simulink model "heli_q8_4_emmerich"  (R2020b)
settings: Solver=ode1  StartTime=0.0  StopTime=inf  FixedStep=0.002  RelTol=1e-3  EnableMultiTasking=on
PostLoadFcn:
  | qc_set_target_type(getConfigSet(bdroot, 'QUARC Default Target Configuration'));
values from neighbouring files (symbols this model uses):
  Ad = eye(6) + T*A + 1/factorial(2)*T^2*A^2 + 1/factorial(3)*T^3*A^3    [init_lab_4.m]
  Bd = (T*eye(6) + 1/factorial(2)*A*T^2 + 1/factorial(3)*A^2*T^3 + 1/factorial(4)*A^3*T^4)*B    [init_lab_4.m]
  Cd = [1 0 0 0 0 0 ... (first row only)    [init_lab_4.m]
  P_init = zeros(6)    [init_lab_4.m]
  Qd = 1000*eye(6)    [init_lab_4.m]
  Rd_move = cov(data_move')    [init_lab_4.m]
  x_init = zeros(6, 1)    [init_lab_4.m]
undefined symbols (not defined in the file or in its folder): F, HIL, Joystick_gain_x, Joystick_gain_y, K, qc_get_step_size, vs0
libraries: quarc_library x9
settings Model: SimulationMode=external  ExtModeTrigDuration=5000  Creator=Rchan  LastModifiedBy=tadyrkor
settings SolverCC: PositivePriorityOrder=on
settings DataIOCC: LimitDataPoints=on  SaveFormat=Array  SignalLoggingSaveFormat=ModelDataLogs  ReturnWorkspaceOutputs=off
settings OptimizationCC: ExpressionDepthLimit=2147483647  InitFltsAndDblsToZero=on  LifeSpan=inf
settings DebuggingCC: SaveWithParameterizedLinksMsg=none  UnderspecifiedInitializationDetection=Classic  MergeDetectMultiDrivingBlocksExec=none  SolverPrmCheckMsg=warning  MultiTaskDSMMsg=warning  MultiTaskCondExecSysMsg=none  FcnCallInpInsideContextMsg=warning  AllowSymbolicDim=off  StateNameClashWarn=warning  SFUnexpectedBacktrackingDiag=warning  SFNoUnconditionalDefaultTransitionDiag=warning  SFExecutionAtInitializationDiag=none  ArithmeticOperatorsInVariantConditions=warning
settings HardwareCC: ProdBitPerPointer=32  ProdBitPerSizeT=32  ProdBitPerPtrDiffT=32  ProdLargestAtomicFloat=None  ProdIntDivRoundTo=Undefined  ProdEndianess=Unspecified  ProdWordSize=32  ProdHWDeviceType=32-bit Generic
settings ModelReferenceCC: PropagateSignalLabelsOutOfModel=off
settings SFSimCC: SimUseLocalCustomCode=off  CustomCodeUndefinedFunction=UseInterfaceOnly
settings RTWCC: Description=QUARC Win64 Target  SystemTargetFile=quarc_win64.tlc  TemplateMakefile=quarc_default_tmf  RTWUseLocalCustomCode=off
settings CodeAppCC: StateflowObjectComments=on
settings GRTTargetCC: TargetLangStandard=C89/C90 (ANSI)  ParMdlRefBuildCompliant=off  CompOptLevelCompliant=off  CombineOutputUpdateFcns=off  MatFileLogging=off  GRTInterface=on  UseToolchainInfoCompliant=off  ExtMode=on  ExtModeMexFile=quarc_comm
settings ConfigComp: CovMetricSettings=dw  CovSaveCumulativeToWorkspaceVar=on  CovSaveSingleToWorkspaceVar=on  CovExternalEMLEnable=off  CovSFcnEnable=off

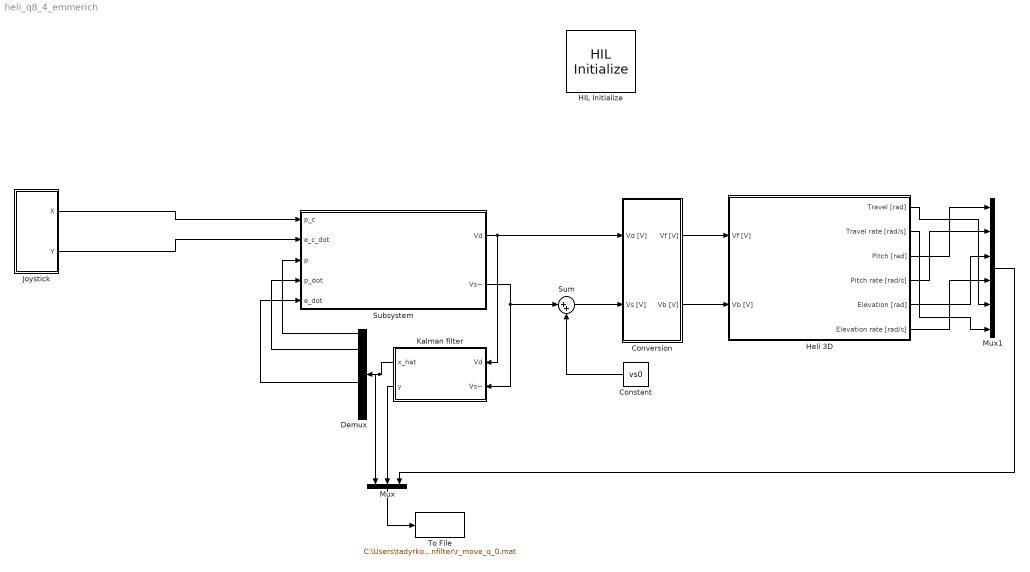
== system heli_q8_4_emmerich ==
  Constant : Constant  Value=vs0
  Conversion : Subsystem
  Demux : Demux  Outputs=6
  HIL Initialize : quarc_library/Data Acquisition/Generic/Configuration/HIL Initialize  Priority=-99  object_name=HIL-1  board_type=q8_usb  board_number=0  board_options=update_rate=normal;decimation=1  exclusive=off  active=off  hardware_clocks=[0:2]  clock_modes=[]  initial_clock_frequencies=[]  set_clock_params_at_start=off  set_clock_params_at_switch_in=off  set_clock_frequencies_at_start=off  set_clock_frequencies_at_switch_in=off  analog_input_channels=[0:7]  analog_input_configurations=[]  analog_input_maximums=10  analog_input_minimums=-10  set_analog_input_params_at_start=on  set_analog_input_params_at_switch_in=off  analog_output_channels=[0:7]  analog_output_maximums=10  analog_output_minimums=-10  initial_analog_outputs=[0]  final_analog_outputs=[0]  watchdog_analog_outputs=0  set_analog_output_params_at_start=on  set_analog_output_params_at_switch_in=off  set_analog_outputs_at_start=on  set_analog_outputs_at_switch_in=off  set_analog_outputs_at_terminate=on  set_analog_outputs_at_switch_out=off  set_analog_outputs_on_watchdog=off  digital_input_channels=[]  digital_output_channels=[]  digital_output_configuration=[]  initial_digital_outputs=[1]  final_digital_outputs=[1]  watchdog_digital_outputs=[1]  set_digital_output_params_at_start=off  set_digital_output_params_at_switch_in=off  set_digital_outputs_at_start=on  set_digital_outputs_at_switch_in=off  set_digital_outputs_at_terminate=on  set_digital_outputs_at_switch_out=off  set_digital_outputs_on_watchdog=off  encoder_channels=[0:7]  quadrature=[4]  encoder_filter_frequency=[]  initial_encoder_counts=[0]  set_encoder_params_at_start=on  set_encoder_params_at_switch_in=off  set_encoder_counts_at_start=on  set_encoder_counts_at_switch_in=off  pwm_channels=[0:7]  pwm_modes=0  pwm_frequency=99.532799999999995e6/4095  pwm_configuration=[0]  pwm_alignment=[0]  pwm_polarity=[1]  pwm_leading_deadband=[0]  pwm_trailing_deadband=[0]  initial_pwm_outputs=[0]  final_pwm_outputs=[0]  watchdog_pwm_outputs=[0]  set_pwm_params_at_start=on  set_pwm_params_at_switch_in=off  set_pwm_outputs_at_start=on  set_pwm_outputs_at_switch_in=off  set_pwm_outputs_at_terminate=on  set_pwm_outputs_at_switch_out=off  set_pwm_outputs_on_watchdog=off  other_output_channels=[]  initial_other_outputs=[]  final_other_outputs=[]  watchdog_other_outputs=[]  set_other_outputs_at_start=off  set_other_outputs_at_switch_in=off  set_other_outputs_at_terminate=off  set_other_outputs_at_switch_out=off  set_other_outputs_on_watchdog=off
  Heli 3D : Subsystem
  Joystick : Subsystem
  Kalman filter : Subsystem
  Mux : Mux  Inputs=3
  Mux1 : Mux  Inputs=6
  Subsystem : Subsystem
  Sum : Sum  Inputs=|++
  To File : ToFile  Filename=C:\Users\tadyrkor\Documents\data\lab4\kalmanfilter\r_move_q_0.mat  MatrixName=measurements
  wires:
  Conversion/2(Vb [V]) -> Heli 3D/2(Vb [V])
  Conversion/1(Vf [V]) -> Heli 3D/1(Vf [V])
  Subsystem/2(Vs~) -> Sum/1, Kalman filter/2(Vs~)
  Subsystem/1(Vd) -> Conversion/1(Vd [V]), Kalman filter/1(Vd)
  Joystick/1(X) -> Subsystem/1(p_c)
  Joystick/2(Y) -> Subsystem/2(e_c_dot)
  Constant/1 -> Sum/2
  Sum/1 -> Conversion/2(Vs [V])
  Kalman filter/1(x_hat) -> Mux/1, Demux/1
  Demux/1 -> Subsystem/3(p)
  Demux/2 -> Subsystem/4(p_dot)
  Demux/4 -> Subsystem/5(e_dot)
  Kalman filter/2(y) -> Mux/2
  Heli 3D/3(Pitch [rad]) -> Mux1/1
  Heli 3D/4(Pitch rate [rad/s]) -> Mux1/2
  Heli 3D/5(Elevation [rad]) -> Mux1/3
  Heli 3D/6(Elevation rate [rad/s]) -> Mux1/4
  Heli 3D/1(Travel [rad]) -> Mux1/5
  Heli 3D/2(Travel rate [rad/s]) -> Mux1/6
  Mux1/1 -> Mux/3
  Mux/1 -> To File/1

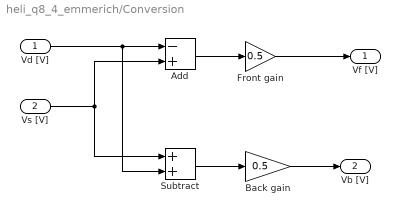
== system heli_q8_4_emmerich/Conversion ==
  Vd [V] : Inport
  Vs [V] : Inport  Port=2
  Add : Sum  Inputs=-+
  Back gain : Gain  Gain=0.5
  Front gain : Gain  Gain=0.5
  Subtract : Sum
  Vf [V] : Outport
  Vb [V] : Outport  Port=2
  wires:
  Vd [V]/1 -> Subtract/2, Add/1
  Vs [V]/1 -> Subtract/1, Add/2
  Subtract/1 -> Back gain/1
  Back gain/1 -> Vb [V]/1
  Add/1 -> Front gain/1
  Front gain/1 -> Vf [V]/1

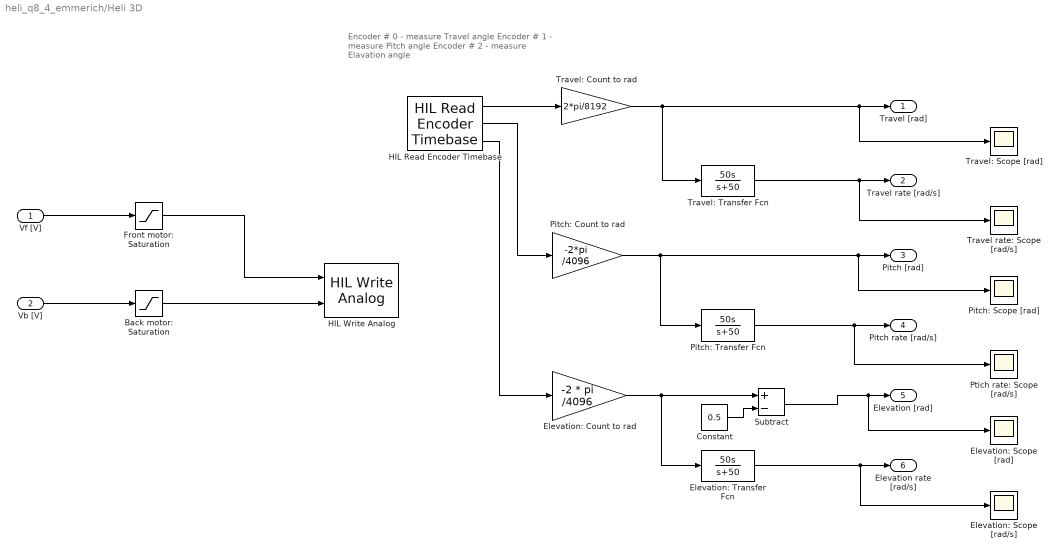
== system heli_q8_4_emmerich/Heli 3D ==
  note: Encoder # 0 - measure Travel angle
      | Encoder # 1 - measure Pitch angle
      | Encoder # 2 - measure Elavation angle
  Vf [V] : Inport
  Vb [V] : Inport  Port=2
  Back motor: Saturation : Saturate  UpperLimit=5  LowerLimit=-5
  Constant : Constant  Value=0.5
  Elevation: Count to rad : Gain  Gain=-2 * pi /4096
  Elevation: Scope [rad/s] : Scope
  Elevation: Scope [rad] : Scope
  Elevation: Transfer Fcn : TransferFcn  Numerator=[50 0]  Denominator=[1 50]
  Front motor: Saturation : Saturate  UpperLimit=5  LowerLimit=-5
  HIL Read Encoder Timebase : quarc_library/Data Acquisition/Generic/Timebases/HIL Read Encoder Timebase  object_name=HIL-1  clock=0  channels=[0:2]  active=on  vector_output=off  data_type_mode=Inherit via back propagation  data_type=double  overflow_mode=Error on overflow  samples_in_buffer=max(ceil(1/qc_get_step_size), 1)
  HIL Write Analog : quarc_library/Data Acquisition/Generic/Immediate I//O/HIL Write Analog  object_name=HIL-1  channels=[0:1]  sample_time=-1  active=off  vector_input=off
  Pitch: Count to rad : Gain  Gain=-2*pi /4096
  Pitch: Scope [rad] : Scope
  Pitch: Transfer Fcn : TransferFcn  Numerator=[50 0]  Denominator=[1 50]
  Ptich rate: Scope [rad/s] : Scope
  Subtract : Sum  Inputs=+-
  Travel rate: Scope [rad/s] : Scope
  Travel: Count to rad : Gain  Gain=2*pi/8192
  Travel: Scope [rad] : Scope
  Travel: Transfer Fcn : TransferFcn  Numerator=[50 0]  Denominator=[1 50]
  Travel [rad] : Outport
  Travel rate [rad/s] : Outport  Port=2
  Pitch [rad] : Outport  Port=3
  Pitch rate [rad/s] : Outport  Port=4
  Elevation [rad] : Outport  Port=5
  Elevation rate [rad/s] : Outport  Port=6
  wires:
  HIL Read Encoder Timebase/1 -> Travel: Count to rad/1
  HIL Read Encoder Timebase/2 -> Pitch: Count to rad/1
  HIL Read Encoder Timebase/3 -> Elevation: Count to rad/1
  Travel: Count to rad/1 -> Travel: Scope [rad]/1, Travel [rad]/1, Travel: Transfer Fcn/1
  Travel: Transfer Fcn/1 -> Travel rate: Scope [rad/s]/1, Travel rate [rad/s]/1
  Pitch: Count to rad/1 -> Pitch: Transfer Fcn/1, Pitch: Scope [rad]/1, Pitch [rad]/1
  Pitch: Transfer Fcn/1 -> Ptich rate: Scope [rad/s]/1, Pitch rate [rad/s]/1
  Elevation: Count to rad/1 -> Subtract/1, Elevation: Transfer Fcn/1
  Elevation: Transfer Fcn/1 -> Elevation: Scope [rad/s]/1, Elevation rate [rad/s]/1
  Vf [V]/1 -> Front motor: Saturation/1
  Vb [V]/1 -> Back motor: Saturation/1
  Front motor: Saturation/1 -> HIL Write Analog/1
  Back motor: Saturation/1 -> HIL Write Analog/2
  Subtract/1 -> Elevation: Scope [rad]/1, Elevation [rad]/1
  Constant/1 -> Subtract/2

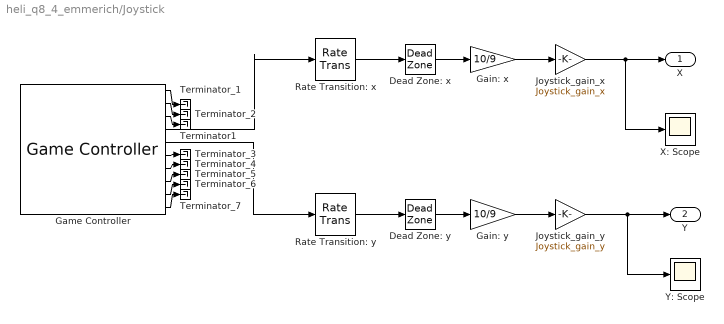
== system heli_q8_4_emmerich/Joystick ==
  Dead Zone: x : DeadZone  LowerValue=-0.1  UpperValue=0.1  SaturateOnIntegerOverflow=on
  Dead Zone: y : DeadZone  LowerValue=-0.1  UpperValue=0.1  SaturateOnIntegerOverflow=on
  Gain: x : Gain  Gain=10/9
  Gain: y : Gain  Gain=10/9
  Game Controller : quarc_library/Devices/Peripherals/Target/Game Controller  controller=1  buffer_size=12  deadzone=[]  saturation=[]  sample_time=max(qc_get_step_size, 0.01)  auto_center=off  enabled=on
      settings: SourceProductName=QUARC Targets
  Joystick_gain_x : Gain  Gain=Joystick_gain_x
  Joystick_gain_y : Gain  Gain=Joystick_gain_y
  Rate Transition: x : RateTransition
  Rate Transition: y : RateTransition
  Terminator1 : Terminator
  Terminator_{1..7} (7 alike) : Terminator
  X: Scope : Scope
  Y: Scope : Scope
  X : Outport
  Y : Outport  Port=2
  wires:
  Rate Transition: y/1 -> Dead Zone: y/1
  Rate Transition: x/1 -> Dead Zone: x/1
  Game Controller/5 -> Rate Transition: y/1
  Game Controller/4 -> Rate Transition: x/1
  Game Controller/1 -> Terminator_1/1
  Game Controller/2 -> Terminator_2/1
  Game Controller/7 -> Terminator_4/1
  Game Controller/8 -> Terminator_5/1
  Game Controller/9 -> Terminator_6/1
  Game Controller/10 -> Terminator_7/1
  Game Controller/3 -> Terminator1/1
  Dead Zone: x/1 -> Gain: x/1
  Dead Zone: y/1 -> Gain: y/1
  Gain: x/1 -> Joystick_gain_x/1
  Gain: y/1 -> Joystick_gain_y/1
  Joystick_gain_x/1 -> X/1, X: Scope/1
  Joystick_gain_y/1 -> Y: Scope/1, Y/1
  Game Controller/6 -> Terminator_3/1

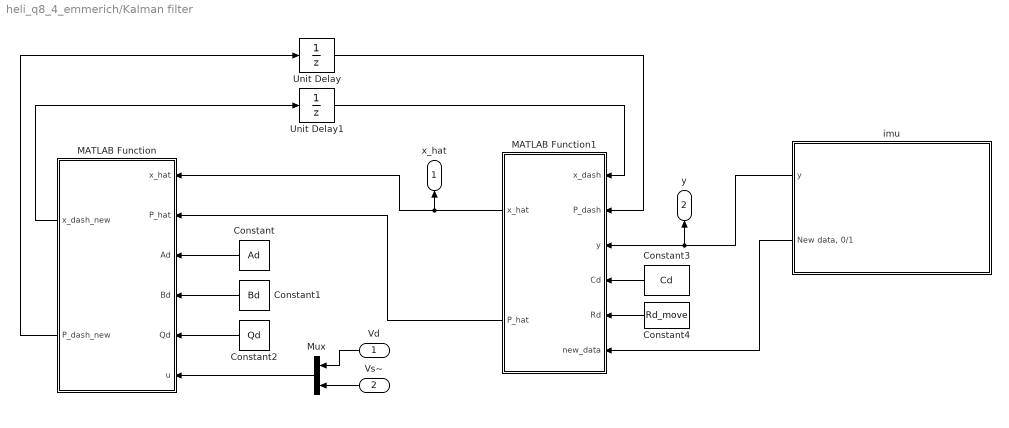
== system heli_q8_4_emmerich/Kalman filter ==
  Vd : Inport
  Vs~ : Inport  Port=2
  Constant : Constant  Value=Ad
  Constant1 : Constant  Value=Bd
  Constant2 : Constant  Value=Qd
  Constant3 : Constant  Value=Cd
  Constant4 : Constant  Value=Rd_move
  MATLAB Function : MATLAB Function  TreatAsAtomicUnit=on
  MATLAB Function1 : MATLAB Function  TreatAsAtomicUnit=on
  Mux : Mux  Inputs=2
  Unit Delay : UnitDelay  InitialCondition=P_init  SampleTime=-1  HasFrameUpgradeWarning=on
  Unit Delay1 : UnitDelay  InitialCondition=x_init  SampleTime=-1  HasFrameUpgradeWarning=on
  imu : Subsystem
  x_hat : Outport
  y : Outport  Port=2
  wires:
  Vs~/1 -> Mux/2
  Vd/1 -> Mux/1
  Mux/1 -> MATLAB Function/6(u)
  imu/1(y) -> MATLAB Function1/3(y), y/1
  imu/2("New data, 0/1") -> MATLAB Function1/6(new_data)
  MATLAB Function1/2(P_hat) -> MATLAB Function/2(P_hat)
  Constant/1 -> MATLAB Function/3(Ad)
  Constant2/1 -> MATLAB Function/5(Qd)
  Constant1/1 -> MATLAB Function/4(Bd)
  Constant3/1 -> MATLAB Function1/4(Cd)
  Constant4/1 -> MATLAB Function1/5(Rd)
  MATLAB Function/1(x_dash_new) -> Unit Delay1/1
  MATLAB Function/2(P_dash_new) -> Unit Delay/1
  Unit Delay/1 -> MATLAB Function1/2(P_dash)
  Unit Delay1/1 -> MATLAB Function1/1(x_dash)
  MATLAB Function1/1(x_hat) -> x_hat/1, MATLAB Function/1(x_hat)

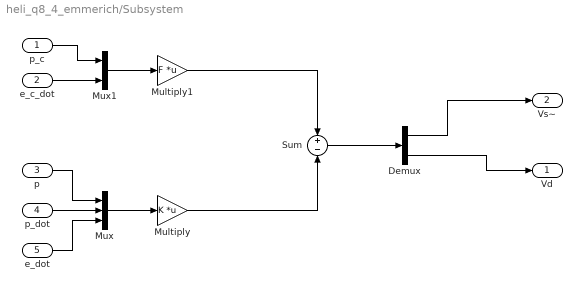
== system heli_q8_4_emmerich/Subsystem ==
  p_c : Inport
  e_c_dot : Inport  Port=2
  p : Inport  Port=3
  p_dot : Inport  Port=4
  e_dot : Inport  Port=5
  Demux : Demux  Outputs=2
  Multiply : Gain  Gain=K  Multiplication=Matrix(K*u)
  Multiply1 : Gain  Gain=F  Multiplication=Matrix(K*u)
  Mux : Mux  Inputs=3
  Mux1 : Mux  Inputs=2
  Sum : Sum  Inputs=+|-
  Vd : Outport
  Vs~ : Outport  Port=2
  wires:
  p/1 -> Mux/1
  p_dot/1 -> Mux/2
  e_dot/1 -> Mux/3
  p_c/1 -> Mux1/1
  e_c_dot/1 -> Mux1/2
  Mux/1 -> Multiply/1
  Sum/1 -> Demux/1
  Multiply/1 -> Sum/2
  Mux1/1 -> Multiply1/1
  Multiply1/1 -> Sum/1
  Demux/1 -> Vs~/1
  Demux/2 -> Vd/1

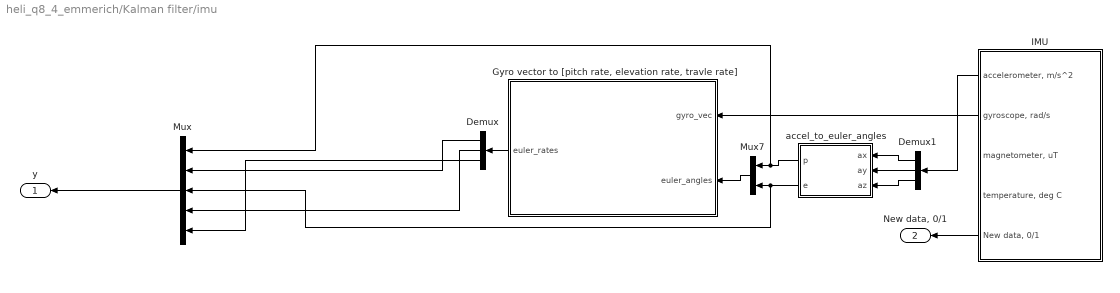
== system heli_q8_4_emmerich/Kalman filter/imu ==
  Demux : Demux  Outputs=3
  Demux1 : Demux  Outputs=3
  "Gyro vector to [pitch rate, elevation rate, travle rate]" : MATLAB Function  TreatAsAtomicUnit=on
  IMU : Subsystem
  Mux : Mux  Inputs=5
  Mux7 : Mux  Inputs=2
  accel_to_euler_angles : MATLAB Function  TreatAsAtomicUnit=on
  y : Outport
  "New data, 0/1" : Outport  Port=2
  wires:
  Mux7/1 -> "Gyro vector to [pitch rate, elevation rate, travle rate]"/2(euler_angles)
  IMU/2("gyroscope, rad/s") -> "Gyro vector to [pitch rate, elevation rate, travle rate]"/1(gyro_vec)
  IMU/1("accelerometer, m/s^2") -> Demux1/1
  accel_to_euler_angles/2(e) -> Mux/3, Mux7/2
  Demux1/1 -> accel_to_euler_angles/1(ax)
  Demux1/3 -> accel_to_euler_angles/3(az)
  accel_to_euler_angles/1(p) -> Mux/1, Mux7/1
  Demux1/2 -> accel_to_euler_angles/2(ay)
  "Gyro vector to [pitch rate, elevation rate, travle rate]"/1(euler_rates) -> Demux/1
  Demux/1 -> Mux/2
  Demux/2 -> Mux/4
  Mux/1 -> y/1
  IMU/5("New data, 0/1") -> "New data, 0/1"/1
  Demux/3 -> Mux/5

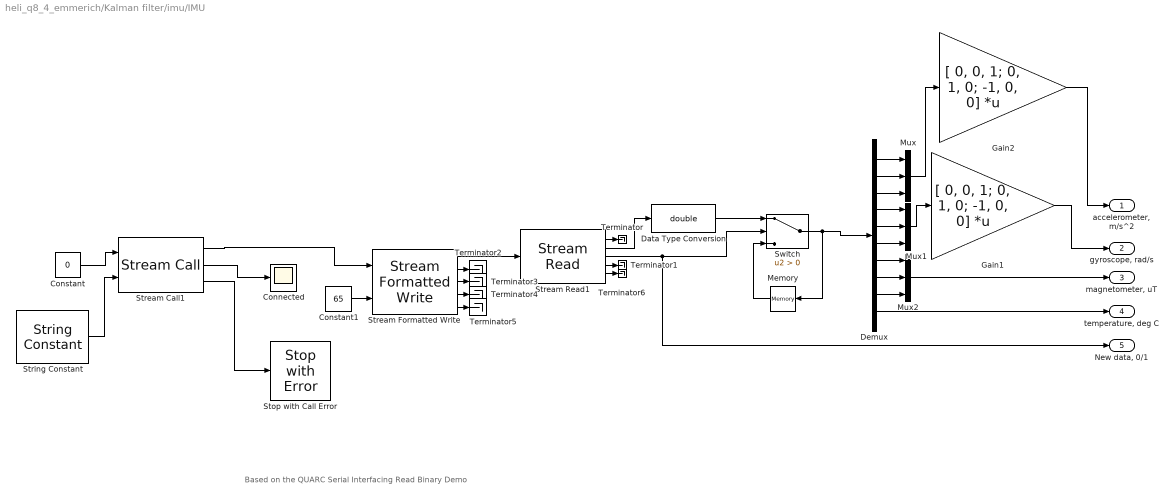
== system heli_q8_4_emmerich/Kalman filter/imu/IMU ==
  note: Based on the QUARC Serial Interfacing Read Binary Demo
  Connected : Scope
  Constant : Constant  Value=0
  Constant1 : Constant  Value=65
  Data Type Conversion : DataTypeConversion  OutDataTypeStr=double
  Demux : Demux  Outputs=10
  Gain1 : Gain  Gain=[ 0, 0, 1; 0, 1, 0; -1, 0, 0]  Multiplication=Matrix(K*u) (u vector)
  Gain2 : Gain  Gain=[ 0, 0, 1; 0, 1, 0; -1, 0, 0]  Multiplication=Matrix(K*u) (u vector)
  Memory : Memory  InitialCondition=[0 0 0 0 0 0 0 0 0 0]
  Mux : Mux  Inputs=3
  Mux1 : Mux  Inputs=3
  Mux2 : Mux  Inputs=3
  Stop with Call Error : quarc_library/Sinks/Error Handling/Stop with Error  message_type=Interpret input as error code  message=Error occurred
      settings: SourceProductName=QUARC Targets
  Stream Call1 : quarc_library/Communications/Intermediate/Stream Call  uri_source=External input port  uri=serial://IMU:9?baud=115200,word=8,parity=none,stop=1,flow='none'  apply_uri_to_all_configs=on  send_buffer_size=8000  receive_buffer_size=8000  byte_order=little endian (Intel - LSB first)  sample_time=qc_get_step_size  non_blocking=on  active=off
      settings: SourceProductName=QUARC Targets
  Stream Formatted Write : quarc_library/Communications/Intermediate/Stream Formatted Write  format_string=%c\n  max_code_units=80  optimization=Minimizing latency
      settings: SourceProductName=QUARC Targets
  Stream Read1 : quarc_library/Communications/Intermediate/Stream Read  data_type=single  type_expr=BusObject  num_elements=10  receive_dims=off
      settings: SourceProductName=QUARC Targets
  String Constant : quarc_library/Strings/String Constant  string_value=qc_perform_substitutions('serial://IMU:%{PORT}?baud=115200,word=8,parity=none,stop=1')  evaluate_string=on  string_type=URI  max_length=255  sample_time=inf  variable_size=off
      settings: AttributesFormatString="\"serial://IMU:5?baud=115200,word=8,parity=none,stop=1\""  SourceProductName=QUARC Targets
  Switch : Switch  Criteria=u2 > Threshold
  Terminator{,1..6} (7 alike) : Terminator
  "accelerometer, m/s^2" : Outport
  "gyroscope, rad/s" : Outport  Port=2
  "magnetometer, uT" : Outport  Port=3
  "temperature, deg C" : Outport  Port=4
  "New data, 0/1" : Outport  Port=5
  wires:
  Switch/1 -> Memory/1, Demux/1
  Data Type Conversion/1 -> Switch/1
  Stream Read1/3 -> "New data, 0/1"/1, Switch/2
  Stream Formatted Write/1 -> Stream Read1/1
  Constant1/1 -> Stream Formatted Write/2
  Gain1/1 -> "gyroscope, rad/s"/1
  Gain2/1 -> "accelerometer, m/s^2"/1
  Stream Read1/4 -> Terminator1/1
  Demux/10 -> "temperature, deg C"/1
  Mux1/1 -> Gain1/1
  Stream Read1/2 -> Data Type Conversion/1
  Demux/7 -> Mux2/1
  Demux/8 -> Mux2/2
  Demux/9 -> Mux2/3
  Mux2/1 -> "magnetometer, uT"/1
  Demux/6 -> Mux1/3
  Demux/5 -> Mux1/2
  Demux/4 -> Mux1/1
  Mux/1 -> Gain2/1
  Demux/3 -> Mux/3
  Demux/1 -> Mux/1
  Demux/2 -> Mux/2
  Stream Read1/1 -> Terminator/1
  Stream Call1/1 -> Stream Formatted Write/1
  Constant/1 -> Stream Call1/1
  String Constant/1 -> Stream Call1/2
  Stream Call1/2 -> Connected/1
  Stream Call1/3 -> Stop with Call Error/1
  Memory/1 -> Switch/3
  Stream Formatted Write/2 -> Terminator2/1
  Stream Formatted Write/3 -> Terminator3/1
  Stream Formatted Write/4 -> Terminator4/1
  Stream Formatted Write/5 -> Terminator5/1
  Stream Read1/5 -> Terminator6/1

== matlab function heli_q8_4_emmerich/Kalman filter/imu/Gyro vector to [pitch rate, elevation rate, travle rate] ==
  data: gyro_vec input; euler_rates output; euler_angles input
function euler_rates = gyro_vec_to_euler_rates(gyro_vec,euler_angles)
%#codegen
phi = euler_angles(1);
theta = euler_angles(2);


T = [1, sin(phi)*tan(theta), cos(phi)*tan(theta);
     0, cos(phi),            -sin(phi);
     0, sin(phi)/cos(theta), cos(phi)/cos(theta)]; 
 
euler_rates = T*gyro_vec;

== matlab function heli_q8_4_emmerich/Kalman filter/imu/accel_to_euler_angles ==
  data: ax input; p output; ay input; az input; e output
function [p, e]  = fcn(ax, ay, az)

if az == 0
    az = 0.1;
end

p = atan(ay/az);


if ay == 0 && az == 0
    ay = 0.1;
    az = 0.1;
end
    
e = atan(ax/sqrt(ay^2 + az^2));

== matlab function heli_q8_4_emmerich/Kalman filter/MATLAB Function ==
  data: x_hat input; P_hat input; Ad input; Bd input; Qd input; u input; x_dash_new output; P_dash_new output
function [x_dash_new, P_dash_new] = prediction_step(x_hat, P_hat, Ad, Bd, Qd, u)

x_dash_new = Ad * x_hat + Bd * u;
P_dash_new = Ad * P_hat * Ad' + Qd;
end

== matlab function heli_q8_4_emmerich/Kalman filter/MATLAB Function1 ==
  data: x_dash input; x_hat output; P_dash input; y input; Cd input; Rd input; new_data input; P_hat output
function [x_hat, P_hat] = correction_step(x_dash, P_dash, y, Cd, Rd, new_data)
    if new_data  % Check if new measurement data is available
        % Kalman gain
        L_kal = P_dash* Cd' * (Cd * P_dash* Cd' + Rd)^(-1);               
        
        % State update
        x_hat = x_dash + L_kal * (y - Cd * x_dash); 
        
        % Covariance update
        P_hat = (eye(size(P_dash)) - L_kal * Cd) * P_dash * (eye(size(P_dash)) - L_kal * Cd)' + L_kal*Rd*L_kal';
    else
        % Initialize outputs
        x_hat = x_dash;
        P_hat = P_dash;
    end
end
